simulink model "Irs"  (Simulink 7.5)
settings: Solver=ode45  StartTime=0.0  StopTime=10.0  RelTol=1e-3
settings Model: Creator=dell  LastModifiedBy=dell

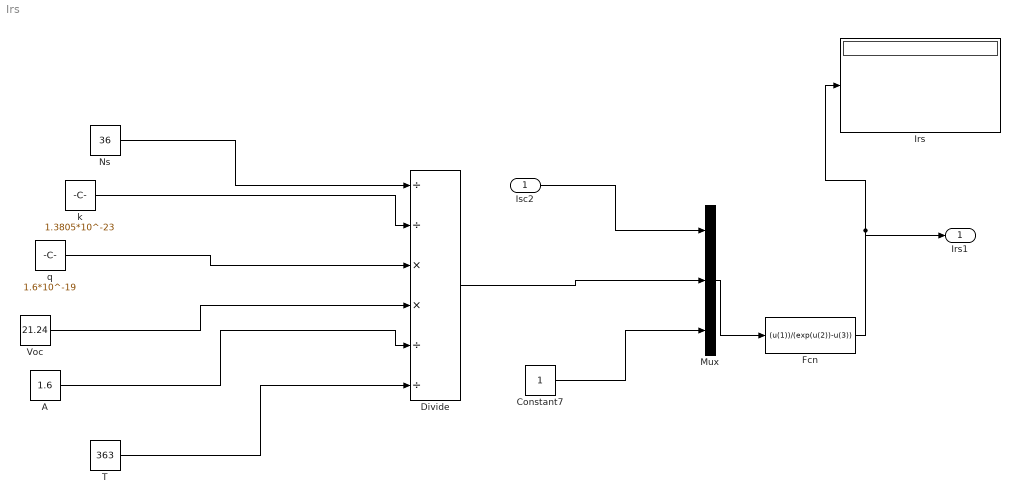
== system Irs ==
  Isc2 : Inport  OutDataType=fixdt(1, 16)  OutScaling=2^0
  A : Constant  Value=1.6  OutDataType=fixdt(1, 16)  OutScaling=2^0
  Constant7 : Constant  OutDataType=fixdt(1, 16)  OutScaling=2^0
  Divide : Product  Inputs=//**//  OutDataType=fixdt(1, 16)  OutScaling=2^-10
  Fcn : Fcn  Expr=(u(1))/(exp(u(2))-u(3))
  Irs : Display
      settings: Format=short_e
  Mux : Mux  Inputs=3
  Ns : Constant  Value=36  OutDataType=fixdt(1, 16)  OutScaling=2^0
  T : Constant  Value=363  OutDataType=fixdt(1, 16)  OutScaling=2^0
  Voc : Constant  Value=21.24  OutDataType=fixdt(1, 16)  OutScaling=2^0
  k : Constant  Value=1.3805*10^-23  OutDataType=fixdt(1, 16)  OutScaling=2^0
  q : Constant  Value=1.6*10^-19  OutDataType=fixdt(1, 16)  OutScaling=2^0
  Irs1 : Outport  OutDataType=fixdt(1, 16)  OutScaling=2^0
  wires:
  Ns/1 -> Divide/1
  k/1 -> Divide/2
  q/1 -> Divide/3
  Voc/1 -> Divide/4
  A/1 -> Divide/5
  T/1 -> Divide/6
  Isc2/1 -> Mux/1
  Divide/1 -> Mux/2
  Mux/1 -> Fcn/1
  Fcn/1 -> Irs/1, Irs1/1
  Constant7/1 -> Mux/3
